simulink model "Lab1"  (Simulink 8.8)
settings: Solver=FixedStepAuto  StartTime=0.0  StopTime=20  FixedStep=0.01  MaxStep=10^-3  RelTol=1e-3  EnableMultiTasking=on
settings Model: Creator=student  LastModifiedBy=Admin
settings OptimizationCC: ExpressionDepthLimit=2147483647  InitFltsAndDblsToZero=on
settings DebuggingCC: SaveWithParameterizedLinksMsg=none  SolverPrmCheckMsg=warning
settings GRTTargetCC: TargetFcnLib=ansi_tfl_tmw.mat  GeneratePreprocessorConditionals=Use local settings

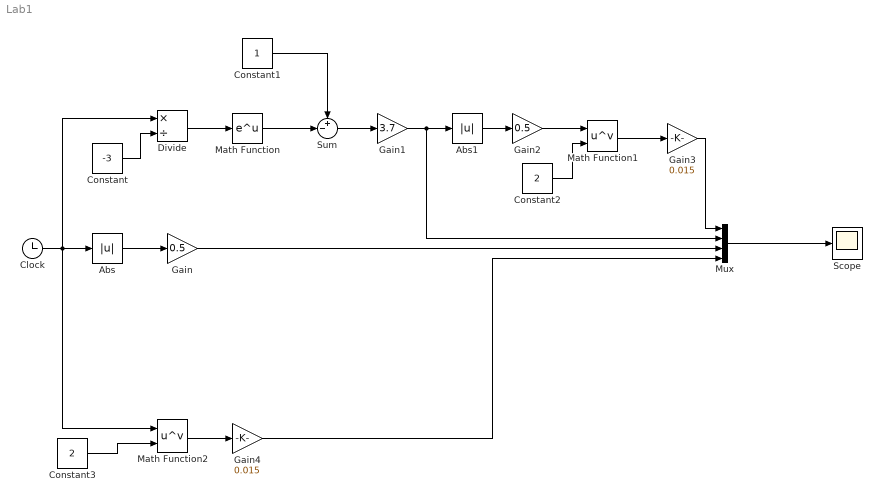
== system Lab1 ==
  Abs : Abs
  Abs1 : Abs
  Clock : Clock
  Constant : Constant  Value=-3
  Constant1 : Constant
  Constant2 : Constant  Value=2
  Constant3 : Constant  Value=2
  Divide : Product  Inputs=*/
  Gain : Gain  Gain=0.5
  Gain1 : Gain  Gain=3.7
  Gain2 : Gain  Gain=0.5
  Gain3 : Gain  Gain=0.015
  Gain4 : Gain  Gain=0.015
  Math Function : Math  SaturateOnIntegerOverflow=on
  Math Function1 : Math  Operator=pow  SaturateOnIntegerOverflow=on
  Math Function2 : Math  Operator=pow  SaturateOnIntegerOverflow=on
  Mux : Mux
  Scope : Scope
  Sum : Sum  Inputs=+-|
  wires:
  Gain1/1 -> Abs1/1, Mux/2
  Divide/1 -> Math Function/1
  Clock/1 -> Divide/1, Abs/1, Math Function2/1
  Constant3/1 -> Math Function2/2
  Abs/1 -> Gain/1
  Constant/1 -> Divide/2
  Constant1/1 -> Sum/1
  Math Function/1 -> Sum/2
  Sum/1 -> Gain1/1
  Abs1/1 -> Gain2/1
  Gain2/1 -> Math Function1/1
  Constant2/1 -> Math Function1/2
  Math Function1/1 -> Gain3/1
  Math Function2/1 -> Gain4/1
  Mux/1 -> Scope/1
  Gain4/1 -> Mux/4
  Gain/1 -> Mux/3
  Gain3/1 -> Mux/1
